simulink model "Bastion"  (R2025b)
settings: Solver=VariableStepAuto  StartTime=0.0  StopTime=1  RelTol=1e-3
libraries: fl_lib x4, nesl_utility x3
settings Model: Creator=PRANAV  LastModifiedBy=PRANAV

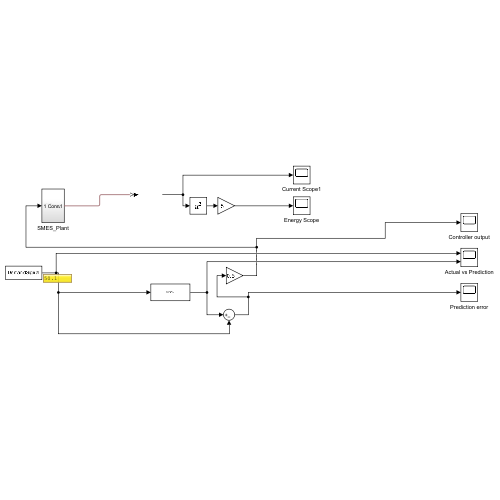
[thumbnail: Simulink's stored preview of the top-level diagram]
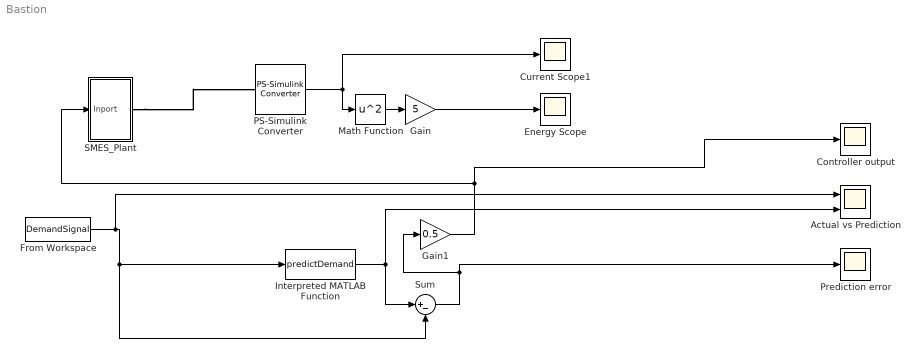
== system Bastion ==
  Actual vs Prediction : Scope  NumInputPorts=2
      settings: ActiveDisplayYMinimum=38.363404037066985  ActiveDisplayYMaximum=74.619001773476072  DataLoggingVariableName=ScopeData3
  Controller output : Scope
      settings: ActiveDisplayYMinimum=-8.0716589334159572  ActiveDisplayYMaximum=8.1346488157299959  DataLoggingVariableName=ScopeData4
  Current Scope1 : Scope
      settings: ActiveDisplayYMinimum=-8.0716589334159572  ActiveDisplayYMaximum=8.1346488157299959
  Energy Scope : Scope
      settings: ActiveDisplayYMinimum=-26.52026888581354  ActiveDisplayYMaximum=238.6824245210266
  From Workspace : FromWorkspace  VariableName=DemandSignal
  Gain : Gain  Gain=5
  Gain1 : Gain  Gain=0.5
  Interpreted MATLAB Function : MATLABFcn  MATLABFcn=predictDemand
  Math Function : Math  Operator=square
  PS-Simulink Converter : nesl_utility/PS-Simulink Converter  PhysicalDomain=network_engine_domain  SubClassName=ps_output  LeftPortType=input  RightPortType=output  PseudoPeriodic=off  Frequencies=[]  VectorFormat=inherit  Unit=inherit  AffineConversion=off
  Prediction error : Scope
      settings: ActiveDisplayYMinimum=-8.2855879704984172  ActiveDisplayYMaximum=12.440001513202297  DataLoggingVariableName=ScopeData2
  SMES_Plant : Subsystem
  Sum : Sum  Inputs=|+-
  wires:
  PS-Simulink Converter/1 -> Current Scope1/1, Math Function/1
  Math Function/1 -> Gain/1
  Gain/1 -> Energy Scope/1
  From Workspace/1 -> Actual vs Prediction/1, Sum/2, Interpreted MATLAB Function/1
  Interpreted MATLAB Function/1 -> Sum/1, Actual vs Prediction/2
  Sum/1 -> Prediction error/1, Gain1/1
  Gain1/1 -> Controller output/1, SMES_Plant/1(Inport)
  connections:
  SMES_Plant/RConn1 -- PS-Simulink Converter/LConn1

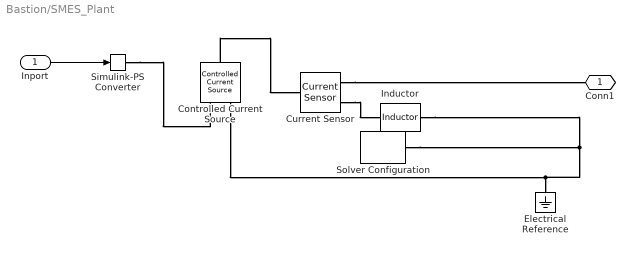
== system Bastion/SMES_Plant ==
  Inport : Inport
  Controlled Current Source : fl_lib/Electrical/Electrical Sources/Controlled Current Source
  Current Sensor : fl_lib/Electrical/Electrical Sensors/Current Sensor
  Electrical Reference : fl_lib/Electrical/Electrical Elements/Electrical Reference
  Inductor : fl_lib/Electrical/Electrical Elements/Inductor  l=10 H  r=0 Ohm  g=1e-9 1/Ohm  i_specify=off  i_priority=None  i=0 A  i_nominal_specify=off  i_nominal_value=1  i_nominal_unit=A  v_specify=off  v_priority=None  v=0 V  v_nominal_specify=off  v_nominal_value=1  v_nominal_unit=V  i_L_specify=off  i_L_priority=High  i_L=0 A  i_L_nominal_specify=off  i_L_nominal_value=1  i_L_nominal_unit=A
  Simulink-PS Converter : nesl_utility/Simulink-PS Converter  PhysicalDomain=network_engine_domain  SubClassName=ps_input  LeftPortType=input  RightPortType=output  PseudoPeriodic=off  Frequencies=[]  NoiseDistribution=none  NoiseParameters=[]  Unit=1  AffineConversion=off  FilteringAndDerivatives=provide  SimscapeFilterOrder=1  InputFilterTimeConstant=0.001  UdotUserProvided=0
  Solver Configuration : nesl_utility/Solver Configuration  PhysicalDomain=network_engine_domain  SubClassName=solver  LeftPortType=input  RightPortType=generic  Tones=[]  Harmonics=[]  SimulateNoise=off  Profile=off  UseLocalSampling=off  EnableSwitchedLinearOptims=on  FrequencyDomain=off  UseCCode=off  RelTol=0.001  AbsTol=0.001  MinStep=1e-09  ToWorkspace=off  RevertToSquareIcSolve=off  NumHomotopyIterations=100  PhasorMode=off  PhasorModeNumHarmonics=1  ConsistencySolver=NEWTON_XTOL_AFTER_FTOL  IndexReductionMethod=DerivativeReplacement  DoDC=off  ResidualTolerance=1e-09  ConsistencyTolSource=GLOBAL  ConsistencyAbsTol=0.001  ConsistencyRelTol=0.001  ConsistencyTolFactor=0.001  UseLocalSolver=off  LocalSolverChoice=NE_BACKWARD_EULER_ADVANCER  ResolveIndetEquations=on  FunctionEvalNumThread=1  LocalSolverSampleTime=0.001  DoFixedCost=off  MaxNonlinIter=3  MaxModeIter=2  ComputeImpulses=off  ImpulseIterations=2  LinearAlgebra=auto  LinearAlgebraNumThread=0  EquationFormulation=NE_TIME_EF  DelaysMemoryBudget=1024  AutomaticFiltering=on  FilteringTimeConstant=0.001  PartitionStorageMethod=AS_NEEDED  PartitionMemoryBudget=1024  PartitionMethod=ROBUST  MultibodyUseLocalSolver=off  MultibodyLocalSolverChoice=ODE1  MultibodyLocalSolverSampleTime=0.001
  Conn1 : PMIOPort  Side=Right
  wires:
  Inport/1 -> Simulink-PS Converter/1
  connections:
  Controlled Current Source/LConn1 -- Current Sensor/LConn1
  Simulink-PS Converter/RConn1 -- Controlled Current Source/RConn1
  Inductor/RConn1 -- Solver Configuration/RConn1 -- Controlled Current Source/RConn2 -- Electrical Reference/LConn1
  Current Sensor/RConn2 -- Inductor/LConn1
  Current Sensor/RConn1 -- Conn1/RConn1
